simulink model "SAD_testControl"  (R2023b)
settings: Solver=ode8  StartTime=0  StopTime=200  FixedStep=t_step  RelTol=1e-3
values from neighbouring files (symbols this model uses):
  A_1 = area_face(1)    [SAD_project_code.m]
  A_2 = area_face(2)    [SAD_project_code.m]
  A_3 = area_face(3)    [SAD_project_code.m]
  A_4 = area_face(4)    [SAD_project_code.m]
  A_5 = area_face(5)    [SAD_project_code.m]
  A_6 = area_face(6)    [SAD_project_code.m]
  DCM_eci_per = rotationMatrix(rad2deg(i),rad2deg(OM), rad2deg(om))    [SAD_project_code.m]
  e = 0.0011241    [SAD_project_code.m]
  FS = 50000e-9    (= 5e-05)    [SAD_project_code.m]
  H0 = [g_10 g_11 h_11]'    [SAD_project_code.m]
  h_r_0 = [0,0,0]'    [SAD_project_code.m]
  horizon_cone_limit = deg2rad(350)    [SAD_project_code.m]
  I = 5/12.*diag([Ix Iy Iz])    [SAD_project_code.m]
  i = deg2rad(97.55)    [SAD_project_code.m]
  I_inv = inv(I)    [SAD_project_code.m]
  I_vector_RW = [I_RW I_RW I_RW]'    [SAD_project_code.m]
  inc_tot = sqrt(inc_lin^2 + inc_acc^2)    [SAD_project_code.m]
  InitialTrueAnomalyOfEarth = 0    [SAD_project_code.m]
  j_b = [0.001 0.005 0.001]'    [SAD_project_code.m]
  K1_point = lqr(A, B, Q, R)    [SAD_project_code.m]
  K2_point = K1_point.^2/2    [SAD_project_code.m]
  matrix_RW_config = eye(3)    [SAD_project_code.m]
  matrix_RW_config_inv = inv(matrix_RW_config)    [SAD_project_code.m]
  mu_E = astroConstants(13)    [SAD_project_code.m]
  N_1 = BODY(1,:)    [SAD_project_code.m]
  N_2 = BODY(2,:)    [SAD_project_code.m]
  N_3 = BODY(3,:)    [SAD_project_code.m]
  N_4 = BODY(4,:)    [SAD_project_code.m]
  N_5 = BODY(5,:)    [SAD_project_code.m]
  N_6 = BODY(6,:)    [SAD_project_code.m]
  n_e = sqrt(mu_E/a^3)    [SAD_project_code.m]
  om = deg2rad(206.3209)    [SAD_project_code.m]
  OM = deg2rad(50.7464)    [SAD_project_code.m]
  p = a*(1-e^2)    [SAD_project_code.m]
  q0 = [0.1, -0.7, 0.51, 0.41]    [SAD_project_code.m]
  r_1 = r(1,:)    [SAD_project_code.m]
  r_2 = r(2,:)    [SAD_project_code.m]
  r_3 = r(3,:)    [SAD_project_code.m]
  r_4 = r(4,:)    [SAD_project_code.m]
  r_5 = r(5,:)    [SAD_project_code.m]
  r_6 = r(6,:)    [SAD_project_code.m]
  R_E = astroConstants(23)    [SAD_project_code.m]
  rho_d1 = 0.1    [SAD_project_code.m]
  rho_d2 = 0.1    [SAD_project_code.m]
  rho_d3 = 0.1    [SAD_project_code.m]
  rho_d4 = 0.1    [SAD_project_code.m]
  rho_d5 = 0.1    [SAD_project_code.m]
  rho_d6 = 0.1    [SAD_project_code.m]
  rho_s1 = rho_s(1)    [SAD_project_code.m]
  rho_s2 = rho_s(2)    [SAD_project_code.m]
  rho_s3 = rho_s(3)    [SAD_project_code.m]
  rho_s4 = rho_s(4)    [SAD_project_code.m]
  rho_s5 = rho_s(5)    [SAD_project_code.m]
  rho_s6 = rho_s(6)    [SAD_project_code.m]
  th0 = deg2rad(0)    [SAD_project_code.m]
  ts_sensor = 5*t_step    (= 0.05)    [SAD_project_code.m]
  w0 = [wx0 wy0 wz0]'    [SAD_project_code.m]
  w0_RW = [0 0 0]    [SAD_project_code.m]
  w_E = deg2rad(15.04)/60/60    [SAD_project_code.m]
  wMax_RW = 2*pi * RPM_max_RW / 60    (= 527.263967027)    [SAD_project_code.m]
libraries: matrix_library x24, simulink_extras x4, sharedtransform x4, simulink x2, vrlib x2, dspfdesign x1, dspinverses x1
(part 3 of 3)

== system SAD_testControl/Enviroment Model/Magnetic Field/Dipol Model of Magnetic Field/Calculation of b_n/m_versor ==
  Clock : Clock
  Constant : Constant  Value=cos(deg2rad(11.5))
  Cos : Trigonometry  Operator=cos
  Gain : Gain  Gain=deg2rad(w_E)
  Gain1 : Gain  Gain=sin(deg2rad(11.5))
  Gain2 : Gain  Gain=sin(deg2rad(11.5))
  Sin : Trigonometry
  Vector Concatenate : Concatenate  NumInputs=3
  m_versor : Outport
  wires:
  Clock/1 -> Gain/1
  Gain/1 -> Sin/1, Cos/1
  Gain2/1 -> Vector Concatenate/2
  Vector Concatenate/1 -> m_versor/1
  Cos/1 -> Gain1/1
  Constant/1 -> Vector Concatenate/3
  Sin/1 -> Gain2/1
  Gain1/1 -> Vector Concatenate/1

== system SAD_testControl/Attitude determination and sensoring/Subsystem/Subsystem/time derivative/Normalize Vector5/Norm vector ==
  Vector : Inport
  Dot Product : DotProduct  OutDataTypeStr=Inherit: Inherit via internal rule
  Sqrt : Sqrt
  Norm : Outport
  wires:
  Sqrt/1 -> Norm/1
  Vector/1 -> Dot Product/1, Dot Product/2
  Dot Product/1 -> Sqrt/1

== system SAD_testControl/Attitude determination and sensoring/Subsystem/Subsystem1/time derivative/Normalize Vector2/Norm vector ==
  Vector : Inport
  Dot Product : DotProduct  OutDataTypeStr=Inherit: Inherit via internal rule
  Sqrt : Sqrt
  Norm : Outport
  wires:
  Sqrt/1 -> Norm/1
  Vector/1 -> Dot Product/1, Dot Product/2
  Dot Product/1 -> Sqrt/1

== system SAD_testControl/Enviroment Model/Magnetic Field/Dipol Model of Magnetic Field/Calculation of b_n/Normalize Vector/Normalize Vector1 ==
  Vector : Inport
  Dot Product : DotProduct  OutDataTypeStr=Inherit: Inherit via internal rule
  Sqrt : Sqrt
  Norm : Outport
  wires:
  Sqrt/1 -> Norm/1
  Vector/1 -> Dot Product/1, Dot Product/2
  Dot Product/1 -> Sqrt/1

== matlab function SAD_testControl/Dynamics e Kinematics/Kinematics quaternion2/MATLAB Function ==
  data: quat input; quat output; quat_last input
function quat = fcn(quat, quat_last)

[~,x] = max(abs(quat_last));  % Pick off index of max abs of last quaternion
if( quat(x)*quat_last(x) < 0 )  % If sign changed ...
    quat = -quat;  % Flip all signs
end

== matlab function SAD_testControl/Determine Control algorithm/DCM to quaternion1/MATLAB Function ==
  data: quat input; quat output; quat_last input
function quat = fcn(quat, quat_last)

[~,x] = max(abs(quat_last));  % Pick off index of max abs of last quaternion
if( quat(x)*quat_last(x) < 0 )  % If sign changed ...
    quat = -quat;  % Flip all signs
end

== matlab function SAD_testControl/DCM to quaternion1/MATLAB Function ==
  data: quat input; quat output; quat_last input
function quat = fcn(quat, quat_last)

[~,x] = max(abs(quat_last));  % Pick off index of max abs of last quaternion
if( quat(x)*quat_last(x) < 0 )  % If sign changed ...
    quat = -quat;  % Flip all signs
end

== matlab function SAD_testControl/Attitude determination and sensoring/Subsystem/DCM to quaternion1/MATLAB Function ==
  data: quat input; quat output; quat_last input
function quat = fcn(quat, quat_last)

[~,x] = max(abs(quat_last));  % Pick off index of max abs of last quaternion
if( quat(x)*quat_last(x) < 0 )  % If sign changed ...
    quat = -quat;  % Flip all signs
end
